simulink model "Active_suspension_Fuzzy_logic"  (R2023a)
settings: Solver=VariableStepAuto  StartTime=0.0  StopTime=10.0  RelTol=1e-3
libraries: fuzblock x1
settings Model: Creator=nanda  LastModifiedBy=nanda

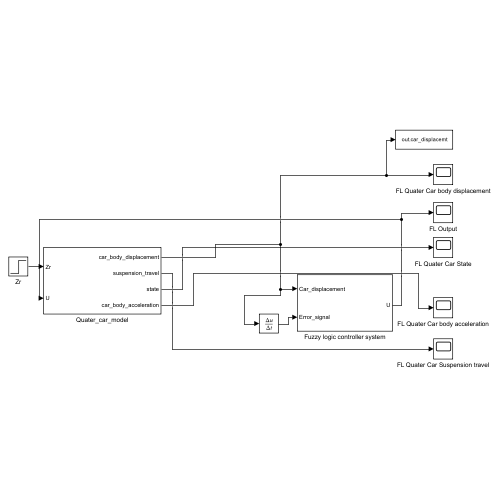
[thumbnail: Simulink's stored preview of the top-level diagram]
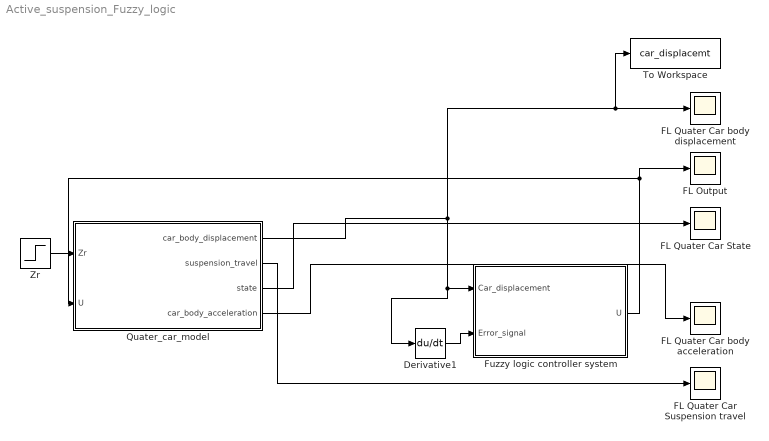
== system Active_suspension_Fuzzy_logic ==
  Derivative1 : Derivative
  FL Output : Scope
  FL Quater Car State : Scope
  FL Quater Car Suspension travel : Scope
  FL Quater Car body acceleration : Scope
  FL Quater Car body displacement : Scope
  Fuzzy logic controller system : Subsystem
  Quater_car_model : Subsystem
  To Workspace : ToWorkspace  VariableName=car_displacemt  SaveFormat=Timeseries  SampleTime=-1
  Zr : Step  After=0.1  SampleTime=0
  wires:
  Quater_car_model/1(car_body_displacement) -> To Workspace/1, FL Quater Car body displacement/1, Derivative1/1, Fuzzy logic controller system/1(Car_displacement)
  Quater_car_model/3(state) -> FL Quater Car State/1
  Quater_car_model/4(car_body_acceleration) -> FL Quater Car body acceleration/1
  Fuzzy logic controller system/1(U) -> Quater_car_model/2(U), FL Output/1
  Derivative1/1 -> Fuzzy logic controller system/2(Error_signal)
  Quater_car_model/2(suspension_travel) -> FL Quater Car Suspension travel/1
  Zr/1 -> Quater_car_model/1(Zr)

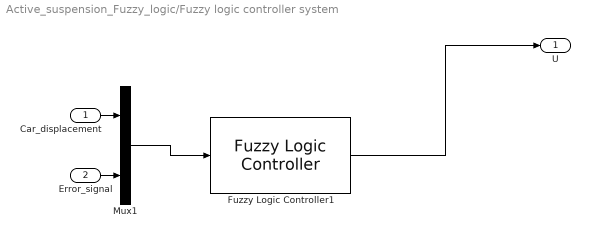
== system Active_suspension_Fuzzy_logic/Fuzzy logic controller system ==
  Car_displacement : Inport
  Error_signal : Inport  Port=2
  Fuzzy Logic Controller1 : fuzblock/Fuzzy Logic  Controller  FIS='Active suspension fuzzy rule.fis'  OutputSampleNumber=101  DataType=double  FuzzifiedInputs=off  RuleFiringStrengths=off  RuleOutputs=off  AggregatedOutputs=off  SimulateUsing=Interpreted execution  OutOfRangeInputValueMessage=warning  NoRuleFiredMessage=warning  EmptyOutputFuzzySetMessage=warning
  Mux1 : Mux  Inputs=2
  U : Outport
  wires:
  Mux1/1 -> Fuzzy Logic Controller1/1
  Car_displacement/1 -> Mux1/1
  Error_signal/1 -> Mux1/2
  Fuzzy Logic Controller1/1 -> U/1

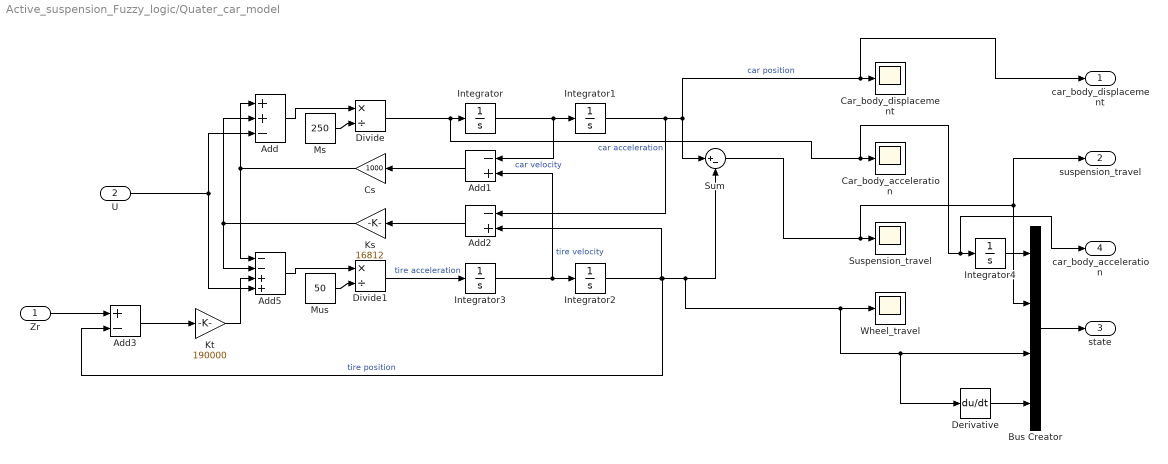
== system Active_suspension_Fuzzy_logic/Quater_car_model ==
  Zr : Inport
  U : Inport  Port=2
  Add : Sum  Inputs=++-
  Add1 : Sum  Inputs=-+
  Add2 : Sum  Inputs=-+
  Add3 : Sum  Inputs=+-
  Add5 : Sum  Inputs=--++
  Bus Creator : BusCreator  Inputs=4
  Car_body_acceleration : Scope
  Car_body_displacement : Scope
  Cs : Gain  Gain=1000
  Derivative : Derivative
  Divide : Product  Inputs=*/
  Divide1 : Product  Inputs=*/
  Integrator{,1..4} (5 alike) : Integrator
  Ks : Gain  Gain=16812
  Kt : Gain  Gain=190000
  Ms : Constant  Value=250
  Mus : Constant  Value=50
  Sum : Sum  Inputs=|+-
  Suspension_travel : Scope
  Wheel_travel : Scope
  car_body_displacement : Outport
  suspension_travel : Outport  Port=2
  state : Outport  Port=3
  car_body_acceleration : Outport  Port=4
  wires:
  Derivative/1 -> Bus Creator/4
  Integrator4/1 -> Bus Creator/1
  Integrator1/1 -> car_body_displacement/1, Car_body_displacement/1, Sum/1, Add2/1  "car position"
  Add1/1 -> Cs/1
  Divide1/1 -> Integrator3/1  "tire acceleration"
  Mus/1 -> Divide1/2
  Integrator3/1 -> Integrator2/1, Add1/2  "tire velocity"
  Sum/1 -> suspension_travel/1, Bus Creator/2, Suspension_travel/1
  Cs/1 -> Add/1, Add5/1
  Divide/1 -> car_body_acceleration/1, Integrator4/1, Car_body_acceleration/1, Integrator/1  "car acceleration"
  Kt/1 -> Add5/3
  Integrator2/1 -> Add3/2, Wheel_travel/1, Derivative/1, Bus Creator/3, Sum/2, Add2/2  "tire position"
  Integrator/1 -> Integrator1/1, Add1/1  "car velocity"
  Ks/1 -> Add5/2, Add/2
  Add2/1 -> Ks/1
  Add5/1 -> Divide1/1
  Add/1 -> Divide/1
  Ms/1 -> Divide/2
  Bus Creator/1 -> state/1
  U/1 -> Add/3, Add5/4
  Add3/1 -> Kt/1
  Zr/1 -> Add3/1
